simulink model "FIR_FILTER"  (R2020a)
settings: Solver=VariableStepAuto  StartTime=0.0  StopTime=10.0  RelTol=1e-3
settings Model: Creator=kasutav  LastModifiedBy=kasutav
settings DataIOCC: SaveOutput=off  SaveTime=off

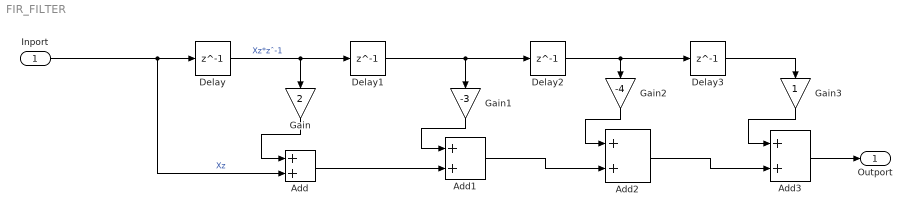
== system FIR_FILTER ==
  Inport : Inport  OutDataTypeStr=double  PortDimensions=1  SampleTime=[0,1]
  Add{,1..3} (4 alike) : Sum
  Delay{,1..3} (4 alike) : Delay  DelayLength=1
  Gain : Gain  Gain=2
  Gain1 : Gain  Gain=-3
  Gain2 : Gain  Gain=-4
  Gain3 : Gain
  Outport : Outport  OutDataTypeStr=double  PortDimensions=1  SampleTime=[0,1]
  wires:
  Gain/1 -> Add/1
  Add2/1 -> Add3/2
  Add/1 -> Add1/2
  Add1/1 -> Add2/2
  Gain1/1 -> Add1/1
  Gain3/1 -> Add3/1
  Delay1/1 -> Delay2/1, Gain1/1
  Delay3/1 -> Gain3/1
  Delay2/1 -> Delay3/1, Gain2/1
  Inport/1 -> Delay/1, Add/2  "Xz"
  Gain2/1 -> Add2/1
  Delay/1 -> Delay1/1, Gain/1  "Xz*zˆ-1"
  Add3/1 -> Outport/1
